simulink model "sampleModel1_pp_1_1"  (R2021b)
settings: Solver=VariableStepAuto  StartTime=0.0  StopTime=10.0  RelTol=1e-3
undefined symbols (not defined in the file or in its folder): DiscIntNeverNeededParam, Newton, Raphson
libraries: simulink x18, slpidlib x4
settings Model: Creator=user  LastModifiedBy=cemery

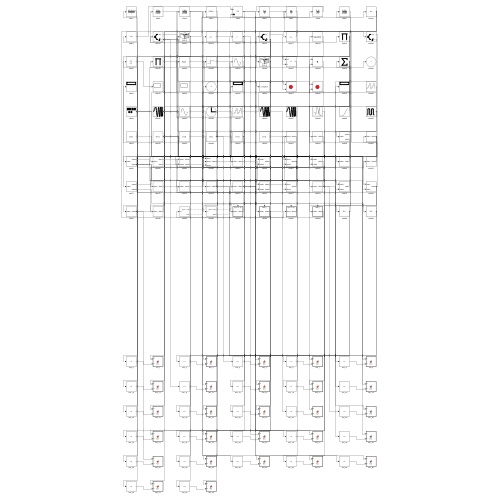
[thumbnail: Simulink's stored preview of the top-level diagram]
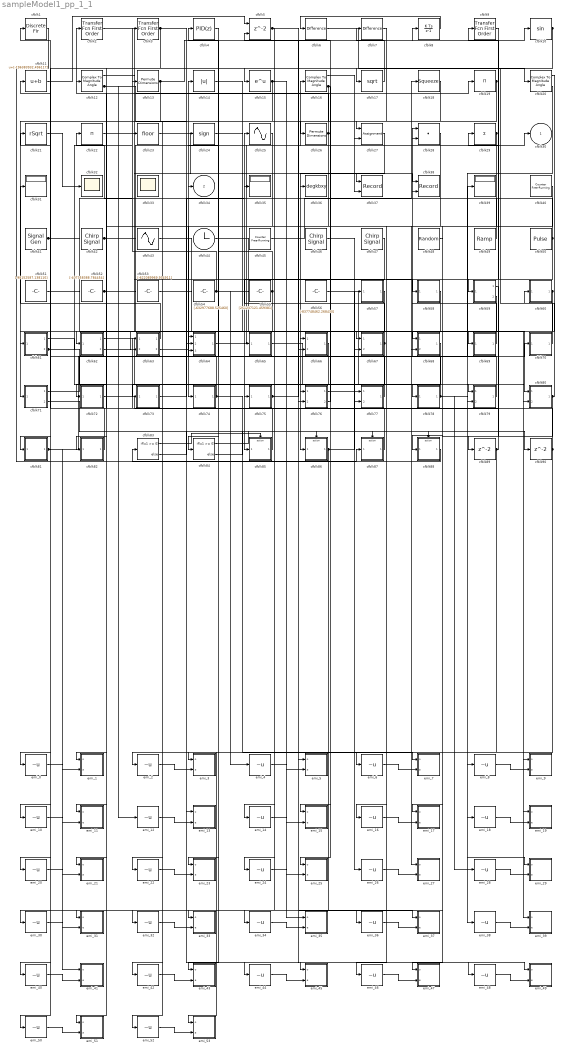
== system sampleModel1_pp_1_1 ==
  cfblk1 : DiscreteFir  SampleTime=1
  cfblk10 : Trigonometry
  cfblk11 : Bias  Bias=[-196383932.496117]
  cfblk12 : ComplexToMagnitudeAngle
  cfblk13 : PermuteDimensions
  cfblk14 : Abs
  cfblk15 : Math  SaturateOnIntegerOverflow=on
  cfblk16 : ComplexToMagnitudeAngle
  cfblk17 : Sqrt  SaturateOnIntegerOverflow=on
  cfblk18 : Squeeze
  cfblk19 : Product  Inputs=*
  cfblk2 : simulink/Discrete/Transfer Fcn First Order  PoleZ=0.95  ICPrevOutput=0.0  DoSatur=off
  cfblk20 : ComplexToMagnitudeAngle
  cfblk21 : Sqrt  Operator=rSqrt  AlgorithmType=Newton-Raphson  SaturateOnIntegerOverflow=on
  cfblk22 : Product  Inputs=*
  cfblk23 : Rounding
  cfblk24 : Signum
  cfblk25 : Sin  TimeSource=Use external signal  SampleTime=0
  cfblk26 : PermuteDimensions
  cfblk27 : Assignment  DiagnosticForDimensions=Warning  IndexOptions=Index vector (dialog)  Indices=1  OutputSizes=1
  cfblk28 : DotProduct  InputSameDT=on  OutDataTypeStr=Inherit: Inherit via internal rule
  cfblk29 : Sum  Inputs=+
  cfblk3 : simulink/Discrete/Transfer Fcn First Order  PoleZ=0.95  ICPrevOutput=0.0  DoSatur=off
  cfblk31 : Display
  cfblk32 : Scope
  cfblk33 : Scope
      settings: Floating=on
  cfblk35 : Display
  cfblk36 : ToWorkspace  VariableName=degkbxy  SaveFormat=Timeseries  SampleTime=-1
  cfblk37 : Record  FileSettingsInternal="{\"entries\":[{\"content\":{\"excelSettings\":{\"content\":{},\"type\":\"Streamout.ExcelSettings\"}},\"type\":\"Streamout.FileSettingStorage\",\"uuid\":\"343f84db-81de-408b-b1a6-f489dfd9fe13\"}],\"packageUris\":[\"http://schema.mathworks.com/mf0/streamout_blocks/R2020a\"],\"version\":\"1.0\"}"  Layout=[1 1]  SignalsInternal="{\"entries\":[{\"content\":{\"signals\":[{\"content\":{\"blockPath\":[\"sampleModel1_pp_1_1/cfblk37\"],\"channel\":[],\"dimensions\":[1],\"domain\":\"sampleModel1_pp_1_1/cfblk37\",\"lineColor\":\"#a2142f\",\"plots\":[],\"port\":1,\"sid\":[\"\"],\"signalID\":352,\"signalName\":\"cfblk14\"},\"type\":\"RecordBlkView.Signal\",\"uuid\":\"d3050f78-5135-48a5-bc90-ebe40b8d4c52\"},{\"content\":{\"blockPath\":[\"sampleModel1_pp_1_1/cfblk37\"],\"channel\":[],\"dimensions\":[1],\"domain\":\"sampleModel1_pp_1_1/cfblk37\",\"lineColor\":\"#139fff\",\"plots\":[],\"port\":2,\"sid\":[\"\"],\"signalID\":356,\"signalName\":\"cfblk16:1\"},\"type\":\"RecordBlkView.Signal\",\"uuid\":\"865a0524-d04f-4987-bc2a-acccf598b7a1\"}]},\"type\":\"RecordBlkView.InputSignals\",\"uuid\":\"039c24d2-93b4-4ea1-bba3-5a71198a0a0e\"}],\"packageUris\":[\"http://schema.mathworks.com/mf0/streamout_blocks/R2020a\"],\"version\":\"1.0\"}"  VisualizationBindings="{\"xyplotplugin\":{\"info\":[{\"series\":[],\"subplotID\":1}]}}"  CompatibilityTag=XY
  cfblk38 : Record  FileSettingsInternal="{\"entries\":[{\"content\":{\"excelSettings\":{\"content\":{},\"type\":\"Streamout.ExcelSettings\"}},\"type\":\"Streamout.FileSettingStorage\",\"uuid\":\"0a5133d1-d1dd-419a-b9c3-011ad09917cf\"}],\"packageUris\":[\"http://schema.mathworks.com/mf0/streamout_blocks/R2020a\"],\"version\":\"1.0\"}"  Layout=[1 1]  SignalsInternal="{\"entries\":[{\"content\":{\"signals\":[{\"content\":{\"blockPath\":[\"sampleModel1_pp_1_1/cfblk38\"],\"channel\":[],\"dimensions\":[1],\"domain\":\"sampleModel1_pp_1_1/cfblk38\",\"lineColor\":\"#ff6929\",\"plots\":[],\"port\":1,\"sid\":[\"\"],\"signalID\":360,\"signalName\":\"cfblk2\"},\"type\":\"RecordBlkView.Signal\",\"uuid\":\"c96adaa5-4d01-4fb0-8fa5-fc7ee38b0bf9\"},{\"content\":{\"blockPath\":[\"sampleModel1_pp_1_1/cfblk38\"],\"channel\":[],\"dimensions\":[1],\"domain\":\"sampleModel1_pp_1_1/cfblk38\",\"lineColor\":\"#b746ff\",\"plots\":[],\"port\":2,\"sid\":[\"\"],\"signalID\":364,\"signalName\":\"cfblk49\"},\"type\":\"RecordBlkView.Signal\",\"uuid\":\"90865e12-c543-48e7-a36c-e57c8157b30f\"}]},\"type\":\"RecordBlkView.InputSignals\",\"uuid\":\"fc363daa-8f32-40cf-99d0-3b294b312640\"}],\"packageUris\":[\"http://schema.mathworks.com/mf0/streamout_blocks/R2020a\"],\"version\":\"1.0\"}"  VisualizationBindings="{\"xyplotplugin\":{\"info\":[{\"series\":[],\"subplotID\":1}]}}"  CompatibilityTag=XY
  cfblk39 : Display
  cfblk4 : slpidlib/PID Controller  Controller=PID  Form=Parallel  TimeDomain=Discrete-time  UseExternalTs=off  SampleTime=1  IntegratorMethod=Forward Euler  FilterMethod=Forward Euler  ControllerParametersSource=internal  P=1  I=1  D=0  UseFilter=on  N=100  TunerSelectOption=Transfer Function Based (PID Tuner App)  InitialConditionSource=internal  InitialConditionForIntegrator=0  InitialConditionForFilter=0  DifferentiatorICPrevScaledInput=0  ExternalReset=none  TrackingMode=off  Kt=1  LimitOutput=off  SatLimitsSource=internal  UpperSaturationLimit=inf  LowerSaturationLimit=-inf  LinearizeAsGain=off  AntiWindupMode=none  Kb=1  POutMin=[]  POutMax=[]  IOutMin=[]  IOutMax=[]  DOutMin=[]  DOutMax=[]  NOutMin=[]  NOutMax=[]  SumOutMin=[]  SumOutMax=[]  SaturationOutMin=[]  SaturationOutMax=[]  PParamMin=[]  PParamMax=[]  IParamMin=[]  IParamMax=[]  DParamMin=[]  DParamMax=[]  NParamMin=[]  NParamMax=[]  KbParamMin=[]  KbParamMax=[]  KtParamMin=[]  KtParamMax=[]  KbOutMin=[]  KbOutMax=[]  KtOutMin=[]  KtOutMax=[]  IntegratorOutMin=[]  IntegratorOutMax=[]  FilterOutMin=[]  FilterOutMax=[]  SumI1OutMin=[]  SumI1OutMax=[]  SumI2OutMin=[]  SumI2OutMax=[]  SumI3OutMin=[]  SumI3OutMax=[]  SumI4OutMin=[]  SumI4OutMax=[]  SumDOutMin=[]  SumDOutMax=[]  DifferentiatorOutMin=[]  DifferentiatorOutMax=[]  FilterDiffOutCoefMin=[]  FilterDiffOutCoefMax=[]  ReciprocalOutMin=[]  ReciprocalOutMax=[]  SumDenOutMin=[]  SumDenOutMax=[]  SumNumOutMin=[]  SumNumOutMax=[]  DivideOutMin=[]  DivideOutMax=[]  UdiffTsProdOutMin=[]  UdiffTsProdOutMax=[]  NTsProdOutMin=[]  NTsProdOutMax=[]  UintegralTsProdOutMin=[]  UintegralTsProdOutMax=[]  UngainTsProdOutMin=[]  UngainTsProdOutMax=[]  IntegratorContinuousStateAttributes=''  IntegratorStateMustResolveToSignalObject=off  IntegratorRTWStateStorageClass=Auto  FilterContinuousStateAttributes=''  FilterStateMustResolveToSignalObject=off  FilterRTWStateStorageClass=Auto  ParallelPVariant=InternalParameters  IdealPVariant=Disabled  IVariant=InternalParameters  DVariant=InternalParameters  IntegratorVariant=Discrete  SatVariant=Disabled  AWVariant=Passthrough  PCopyVariant=Disabled  TRVariant=Disabled  FdbkBlocksVariant=Forward  IdealPFdbkVariant=Disabled  SatFdbkVariant=Disabled  DerivativeFilterVariant=ForwardEulerFilter  NVariant=InternalParameters  NCopyVariant=Disabled  FilterICVariant=InternalICsFilter  IntegratorICVariant=InternalICs  ExternalResetVariant=Disabled  TRSumVariant=Passthrough  SumFdbkVariant=Disabled  SumVariant=Sum_PID  TsampFilterVariant=InternalTs  TsampNgainVariant=Passthrough  TsampIntegralVariant=Passthrough  ExternalSaturationOutDataTypeStr=Inherit: Same as second input
  cfblk40 : simulink/Sources/Counter Free-Running  NumBits=[29.000000]  tsamp=-1
  cfblk41 : SignalGenerator  WaveForm=square  Amplitude=[-21494723.199962]
  cfblk42 : simulink/Sources/Chirp Signal  f1=[-261506437.759570]  T=[-777594489.412425]  f2=[560504136.642276]
  cfblk43 : Sin  Amplitude=[-220522326.077493]  Bias=[-516617428.172335]  SampleTime=0
  cfblk44 : Clock
  cfblk45 : simulink/Sources/Counter Free-Running  NumBits=[24.000000]  tsamp=-1
  cfblk46 : simulink/Sources/Chirp Signal  f1=[-807090949.663223]  T=[-736053414.787330]  f2=[884101181.550970]
  cfblk47 : simulink/Sources/Chirp Signal  f1=[912269080.459605]  T=[150417190.156931]  f2=[-880440914.105688]
  cfblk48 : RandomNumber  Mean=[-53044.017326]  Variance=[35315.857122]  Seed=[821194040.000000]  SampleTime=0.1
  cfblk49 : simulink/Sources/Ramp  slope=[-9691.931247]  start=[3.108166]  InitialOutput=[-662019.941075]
  cfblk5 : Delay  ShowEnablePort=on  SampleTime=1
      settings: InputPortMap=u0,e6
  cfblk50 : DiscretePulseGenerator  PulseType=Time based  Amplitude=[298230949.912904]  Period=[73172238.834145]  PulseWidth=5  PhaseDelay=[6.000000]
  cfblk51 : Constant  Value=[-98152587.138110]  SampleTime=1
  cfblk52 : Constant  Value=[-407358388.784454]  SampleTime=1
  cfblk53 : Constant  Value=[-622089969.934911]  SampleTime=1
  cfblk54 : Constant  Value=[-632977688.525460]  SampleTime=1
  cfblk55 : Constant  Value=[251237121.459381]  SampleTime=1
  cfblk56 : Constant  Value=[-837748462.268430]  SampleTime=1
  cfblk57 : Subsystem
  cfblk58 : Subsystem
  cfblk59 : Subsystem
  cfblk6 : simulink/Discrete/Difference  ICPrevInput=0.0  OutMin=[]  OutMax=[]  OutDataTypeStr=Inherit: Inherit via back propagation  OutDataType=fixdt(1, 16)  OutScaling=2^-10  DoSatur=off
  cfblk60 : Subsystem
  cfblk61 : Subsystem
  cfblk62 : Subsystem
  cfblk63 : Subsystem
  cfblk64 : Subsystem
  cfblk65 : Subsystem
  cfblk66 : Subsystem
  cfblk67 : Subsystem
  cfblk68 : Subsystem
  cfblk69 : Subsystem
  cfblk7 : simulink/Discrete/Difference  ICPrevInput=0.0  OutMin=[]  OutMax=[]  OutDataTypeStr=Inherit: Inherit via back propagation  OutDataType=fixdt(1, 16)  OutScaling=2^-10  DoSatur=off
  cfblk70 : Subsystem
  cfblk71 : Subsystem
  cfblk72 : Subsystem
  cfblk73 : Subsystem
  cfblk74 : Subsystem
  cfblk75 : Subsystem
  cfblk76 : Subsystem
  cfblk77 : Subsystem
  cfblk78 : Subsystem
  cfblk79 : Subsystem
  cfblk8 : DiscreteIntegrator  ICPrevOutput=DiscIntNeverNeededParam  ICPrevScaledInput=DiscIntNeverNeededParam
  cfblk80 : Subsystem
  cfblk81 : Subsystem
  cfblk82 : Subsystem
  cfblk83 : If  IfExpression=u1 >= 0  SampleTime=1
  cfblk84 : If  IfExpression=u1 >= 0  SampleTime=1
  cfblk85 : Subsystem  TreatAsAtomicUnit=on
  cfblk86 : Subsystem  TreatAsAtomicUnit=on
  cfblk87 : Subsystem  TreatAsAtomicUnit=on
  cfblk88 : Subsystem  TreatAsAtomicUnit=on
  cfblk89 : Delay  SampleTime=1
  cfblk9 : simulink/Discrete/Transfer Fcn First Order  PoleZ=0.95  ICPrevOutput=0.0  DoSatur=off
  cfblk90 : Delay  SampleTime=1
  emi_{0,2,4,6,8,10,12,14,16,18,20,22,24,26,28,30,32,34,36,38,40,42,44,46,48,50,52} (27 alike) : UnaryMinus
  emi_1 : MATLAB Function  TreatAsAtomicUnit=on
  emi_11 : MATLAB Function  TreatAsAtomicUnit=on
  emi_13 : MATLAB Function  TreatAsAtomicUnit=on
  emi_15 : MATLAB Function  TreatAsAtomicUnit=on
  emi_17 : MATLAB Function  TreatAsAtomicUnit=on
  emi_19 : MATLAB Function  TreatAsAtomicUnit=on
  emi_21 : MATLAB Function  TreatAsAtomicUnit=on
  emi_23 : MATLAB Function  TreatAsAtomicUnit=on
  emi_25 : MATLAB Function  TreatAsAtomicUnit=on
  emi_27 : MATLAB Function  TreatAsAtomicUnit=on
  emi_29 : MATLAB Function  TreatAsAtomicUnit=on
  emi_3 : MATLAB Function  TreatAsAtomicUnit=on
  emi_31 : MATLAB Function  TreatAsAtomicUnit=on
  emi_33 : MATLAB Function  TreatAsAtomicUnit=on
  emi_35 : MATLAB Function  TreatAsAtomicUnit=on
  emi_37 : MATLAB Function  TreatAsAtomicUnit=on
  emi_39 : MATLAB Function  TreatAsAtomicUnit=on
  emi_41 : MATLAB Function  TreatAsAtomicUnit=on
  emi_43 : MATLAB Function  TreatAsAtomicUnit=on
  emi_45 : MATLAB Function  TreatAsAtomicUnit=on
  emi_47 : MATLAB Function  TreatAsAtomicUnit=on
  emi_49 : MATLAB Function  TreatAsAtomicUnit=on
  emi_5 : MATLAB Function  TreatAsAtomicUnit=on
  emi_51 : MATLAB Function  TreatAsAtomicUnit=on
  emi_53 : MATLAB Function  TreatAsAtomicUnit=on
  emi_7 : MATLAB Function  TreatAsAtomicUnit=on
  emi_9 : MATLAB Function  TreatAsAtomicUnit=on
  cfblk30 : Outport
  cfblk34 : Outport  Port=2
  wires:
  cfblk19/1 -> cfblk71/1(cfblk1), emi_42/1, emi_43/1(o)
  cfblk63/1(cfblk2) -> cfblk31/1
  cfblk67/1(cfblk2) -> cfblk25/1, emi_22/1, emi_23/1(o)
  cfblk62/1(cfblk2) -> cfblk28/1
  cfblk44/1 -> cfblk68/1(cfblk1)
  cfblk26/1 -> cfblk2/1, emi_14/1, emi_15/1(o)
  cfblk21/1 -> cfblk32/1
  cfblk74/1(cfblk2) -> cfblk14/1, emi_6/1, emi_7/1(o)
  cfblk79/1(cfblk2) -> cfblk34/1
  cfblk69/1(cfblk2) -> cfblk28/2
  cfblk72/1(cfblk2) -> cfblk29/1
  cfblk29/1 -> cfblk74/1(cfblk1), emi_46/1, emi_47/1(o)
  cfblk70/1(cfblk2) -> cfblk15/1
  cfblk23/1 -> cfblk86/1(cfblk1)
  cfblk43/1 -> cfblk66/1(cfblk1)
  cfblk65/1(cfblk2) -> cfblk78/1(cfblk1)
  cfblk77/1(cfblk2) -> cfblk11/1
  cfblk48/1 -> cfblk88/1(cfblk1)
  cfblk53/1 -> cfblk80/1(cfblk1)
  cfblk13/1 -> cfblk10/1, emi_0/1, emi_1/1(o)
  cfblk64/1(cfblk2) -> cfblk30/1
  cfblk68/1(cfblk2) -> cfblk76/1(cfblk1)
  cfblk50/1 -> cfblk22/1, emi_16/1, emi_17/1(o)
  cfblk8/1 -> cfblk6/1
  cfblk12/1 -> cfblk58/1(cfblk1)
  cfblk9/1 -> cfblk59/1(cfblk1)
  cfblk78/1(cfblk2) -> cfblk4/1, emi_28/1, emi_29/1(o)
  cfblk85/1(cfblk2) -> cfblk63/1(cfblk1)
  cfblk52/1 -> cfblk69/1(cfblk1), emi_38/1, emi_39/1(o)
  cfblk76/1(cfblk2) -> cfblk77/1(cfblk1)
  cfblk1/1 -> cfblk87/1(cfblk1)
  cfblk56/1 -> cfblk79/1(cfblk1)
  cfblk47/1 -> cfblk85/1(cfblk1)
  cfblk71/1(cfblk2) -> cfblk39/1
  cfblk45/1 -> cfblk18/1
  cfblk51/1 -> cfblk80/2(cfblk3)
  cfblk62/2(cfblk4) -> cfblk76/2(cfblk4)
  cfblk15/1 -> cfblk62/1(cfblk1), emi_34/1, emi_35/1(o)
  cfblk5/1 -> cfblk65/1(cfblk1), emi_36/1, emi_37/1(o)
  cfblk59/2(cfblk3) -> cfblk63/2(cfblk4)
  cfblk81/1(cfblk2) -> cfblk70/1(cfblk1), emi_40/1, emi_41/1(o)
  cfblk66/1(cfblk2) -> cfblk84/1
  cfblk86/1(cfblk2) -> cfblk57/1(cfblk1), emi_30/1, emi_31/1(o)
  cfblk2/1 -> cfblk38/1
  cfblk75/1(cfblk2) -> cfblk8/1, emi_48/1, emi_49/1(o)
  cfblk73/1(cfblk2) -> cfblk35/1
  cfblk42/1 -> cfblk16/1, emi_8/1, emi_9/1(o)
  cfblk4/1 -> cfblk64/1(cfblk1)
  cfblk22/1 -> cfblk64/2(cfblk3)
  cfblk41/1 -> cfblk3/1, emi_26/1, emi_27/1(o)
  cfblk10/1 -> cfblk17/1, emi_10/1, emi_11/1(o)
  cfblk12/2 -> cfblk19/1, emi_12/1, emi_13/1(o)
  cfblk6/1 -> cfblk20/1
  cfblk20/1 -> cfblk67/1(cfblk1)
  cfblk58/1(cfblk2) -> cfblk61/1(cfblk1)
  cfblk49/1 -> cfblk38/2
  cfblk14/1 -> cfblk37/1
  cfblk80/1(cfblk2) -> cfblk60/1(cfblk1), emi_32/1, emi_33/1(o)
  cfblk20/2 -> cfblk79/2(cfblk3)
  cfblk54/1 -> cfblk13/1, emi_4/1, emi_5/1(o)
  cfblk28/1 -> cfblk68/2(cfblk5)
  cfblk87/1(cfblk2) -> cfblk21/1
  cfblk11/1 -> cfblk5/1
  cfblk17/1 -> cfblk7/1
  cfblk57/1(cfblk2) -> cfblk67/2(cfblk4)
  cfblk82/1(cfblk2) -> cfblk1/1
  cfblk61/1(cfblk2) -> cfblk75/1(cfblk1)
  cfblk88/1(cfblk2) -> cfblk83/1
  cfblk60/1(cfblk2) -> cfblk81/1(cfblk1), emi_50/1, emi_51/1(o)
  cfblk16/1 -> cfblk37/2
  cfblk7/1 -> cfblk27/1
  cfblk76/2(cfblk5) -> cfblk5/2
  cfblk18/1 -> cfblk27/2
  cfblk27/1 -> cfblk36/1
  cfblk3/1 -> cfblk72/1(cfblk1), emi_44/1, emi_45/1(o)
  cfblk46/1 -> cfblk77/2(cfblk4)
  cfblk25/1 -> cfblk73/1(cfblk1)
  cfblk16/2 -> cfblk26/1, emi_24/1, emi_25/1(o)
  cfblk61/2(cfblk3) -> cfblk23/1, emi_18/1, emi_19/1(o)
  cfblk63/2(cfblk5) -> cfblk64/3(cfblk4)
  cfblk55/1 -> cfblk24/1, emi_20/1, emi_21/1(o)
  cfblk40/1 -> cfblk82/1(cfblk1)
  cfblk24/1 -> cfblk66/2(cfblk5)
  cfblk83/1 -> cfblk85/Action
  cfblk83/2 -> cfblk86/Action
  cfblk84/1 -> cfblk87/Action
  cfblk84/2 -> cfblk88/Action
  cfblk59/1(cfblk2) -> cfblk89/1
  cfblk89/1 -> cfblk9/1, emi_52/1, emi_53/1(o)
  cfblk71/2(cfblk5) -> cfblk90/1
  cfblk90/1 -> cfblk12/1, emi_2/1, emi_3/1(o)
  emi_0/1 -> emi_1/2(e)
  emi_2/1 -> emi_3/2(e)
  emi_4/1 -> emi_5/2(e)
  emi_6/1 -> emi_7/2(e)
  emi_8/1 -> emi_9/2(e)
  emi_10/1 -> emi_11/2(e)
  emi_12/1 -> emi_13/2(e)
  emi_14/1 -> emi_15/2(e)
  emi_16/1 -> emi_17/2(e)
  emi_18/1 -> emi_19/2(e)
  emi_20/1 -> emi_21/2(e)
  emi_22/1 -> emi_23/2(e)
  emi_24/1 -> emi_25/2(e)
  emi_26/1 -> emi_27/2(e)
  emi_28/1 -> emi_29/2(e)
  emi_30/1 -> emi_31/2(e)
  emi_32/1 -> emi_33/2(e)
  emi_34/1 -> emi_35/2(e)
  emi_36/1 -> emi_37/2(e)
  emi_38/1 -> emi_39/2(e)
  emi_40/1 -> emi_41/2(e)
  emi_42/1 -> emi_43/2(e)
  emi_44/1 -> emi_45/2(e)
  emi_46/1 -> emi_47/2(e)
  emi_48/1 -> emi_49/2(e)
  emi_50/1 -> emi_51/2(e)
  emi_52/1 -> emi_53/2(e)

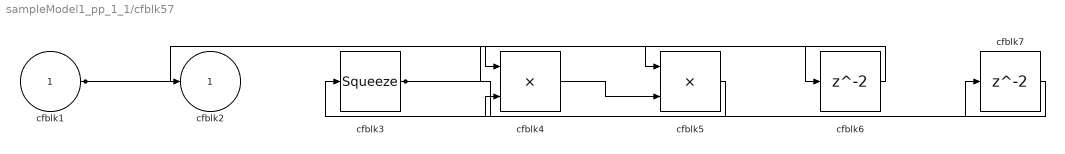
== system sampleModel1_pp_1_1/cfblk57 ==
  cfblk1 : Inport
  cfblk3 : Squeeze
  cfblk4 : Product
  cfblk5 : Product
  cfblk6 : Delay  SampleTime=1
  cfblk7 : Delay  SampleTime=1
  cfblk2 : Outport
  wires:
  cfblk3/1 -> cfblk6/1, cfblk7/1
  cfblk5/1 -> cfblk3/1
  cfblk1/1 -> cfblk4/1, cfblk2/1
  cfblk4/1 -> cfblk5/2
  cfblk6/1 -> cfblk5/1
  cfblk7/1 -> cfblk4/2

== system sampleModel1_pp_1_1/cfblk58 ==
  cfblk1 : Inport
  cfblk3 : DotProduct  InputSameDT=on  OutDataTypeStr=Inherit: Inherit via internal rule
  cfblk2 : Outport
  wires:
  cfblk1/1 -> cfblk3/1, cfblk3/2
  cfblk3/1 -> cfblk2/1

== system sampleModel1_pp_1_1/cfblk59 ==
  cfblk1 : Inport
  cfblk2 : Outport
  cfblk3 : Outport  Port=2
  wires:
  cfblk1/1 -> cfblk2/1, cfblk3/1

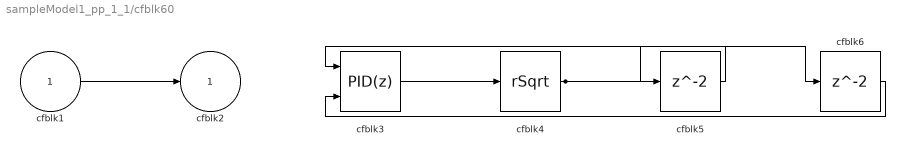
== system sampleModel1_pp_1_1/cfblk60 ==
  cfblk1 : Inport
  cfblk3 : slpidlib/PID Controller (2DOF)  Controller=PID  Form=Parallel  TimeDomain=Discrete-time  UseExternalTs=off  SampleTime=1  IntegratorMethod=Forward Euler  FilterMethod=Forward Euler  ControllerParametersSource=internal  P=1  I=1  D=0  UseFilter=on  N=100  b=1  c=1  TunerSelectOption=Transfer Function Based (PID Tuner App)  InitialConditionSource=internal  InitialConditionForIntegrator=0  InitialConditionForFilter=0  DifferentiatorICPrevScaledInput=0  ExternalReset=none  TrackingMode=off  Kt=1  LimitOutput=off  SatLimitsSource=internal  UpperSaturationLimit=inf  LowerSaturationLimit=-inf  LinearizeAsGain=off  AntiWindupMode=none  Kb=1  POutMin=[]  POutMax=[]  IOutMin=[]  IOutMax=[]  DOutMin=[]  DOutMax=[]  NOutMin=[]  NOutMax=[]  bOutMin=[]  bOutMax=[]  cOutMin=[]  cOutMax=[]  SumOutMin=[]  SumOutMax=[]  SaturationOutMin=[]  SaturationOutMax=[]  PParamMin=[]  PParamMax=[]  IParamMin=[]  IParamMax=[]  DParamMin=[]  DParamMax=[]  NParamMin=[]  NParamMax=[]  bParamMin=[]  bParamMax=[]  cParamMin=[]  cParamMax=[]  KbParamMin=[]  KbParamMax=[]  KtParamMin=[]  KtParamMax=[]  KbOutMin=[]  KbOutMax=[]  KtOutMin=[]  KtOutMax=[]  IntegratorOutMin=[]  IntegratorOutMax=[]  FilterOutMin=[]  FilterOutMax=[]  SumI1OutMin=[]  SumI1OutMax=[]  SumI2OutMin=[]  SumI2OutMax=[]  SumI3OutMin=[]  SumI3OutMax=[]  SumI4OutMin=[]  SumI4OutMax=[]  SumDOutMin=[]  SumDOutMax=[]  Sum1OutMin=[]  Sum1OutMax=[]  Sum2OutMin=[]  Sum2OutMax=[]  Sum3OutMin=[]  Sum3OutMax=[]  DifferentiatorOutMin=[]  DifferentiatorOutMax=[]  FilterDiffOutCoefMin=[]  FilterDiffOutCoefMax=[]  ReciprocalOutMin=[]  ReciprocalOutMax=[]  SumDenOutMin=[]  SumDenOutMax=[]  SumNumOutMin=[]  SumNumOutMax=[]  DivideOutMin=[]  DivideOutMax=[]  UdiffTsProdOutMin=[]  UdiffTsProdOutMax=[]  NTsProdOutMin=[]  NTsProdOutMax=[]  UintegralTsProdOutMin=[]  UintegralTsProdOutMax=[]  UngainTsProdOutMin=[]  UngainTsProdOutMax=[]  IntegratorContinuousStateAttributes=''  IntegratorStateMustResolveToSignalObject=off  IntegratorRTWStateStorageClass=Auto  FilterContinuousStateAttributes=''  FilterStateMustResolveToSignalObject=off  FilterRTWStateStorageClass=Auto  ParallelPVariant=InternalParameters  IdealPVariant=Disabled  IVariant=InternalParameters  DVariant=InternalParameters  bVariant=InternalParameters  cVariant=InternalParameters  IntegratorVariant=Discrete  SatVariant=Disabled  AWVariant=Passthrough  PCopyVariant=Disabled  TRVariant=Disabled  FdbkBlocksVariant=Forward  IdealPFdbkVariant=Disabled  SatFdbkVariant=Disabled  DerivativeFilterVariant=ForwardEulerFilter  NVariant=InternalParameters  NCopyVariant=Disabled  FilterICVariant=InternalICsFilter  IntegratorICVariant=InternalICs  ExternalResetVariant=Disabled  TRSumVariant=Passthrough  SumFdbkVariant=Disabled  SumVariant=Sum_PID  TsampFilterVariant=InternalTs  TsampNgainVariant=Passthrough  TsampIntegralVariant=Passthrough  ExternalSaturationOutDataTypeStr=Inherit: Same as second input
      settings: SourceProductBaseCode=SL
  cfblk4 : Sqrt  Operator=rSqrt  AlgorithmType=Newton-Raphson  SaturateOnIntegerOverflow=on
  cfblk5 : Delay  SampleTime=1
  cfblk6 : Delay  SampleTime=1
  cfblk2 : Outport
  wires:
  cfblk4/1 -> cfblk5/1, cfblk6/1
  cfblk1/1 -> cfblk2/1
  cfblk3/1 -> cfblk4/1
  cfblk5/1 -> cfblk3/1
  cfblk6/1 -> cfblk3/2

== system sampleModel1_pp_1_1/cfblk61 ==
  cfblk1 : Inport
  cfblk2 : Outport
  cfblk3 : Outport  Port=2
  wires:
  cfblk1/1 -> cfblk3/1, cfblk2/1

== system sampleModel1_pp_1_1/cfblk62 ==
  cfblk1 : Inport
  cfblk3 : Product
  cfblk2 : Outport
  cfblk4 : Outport  Port=2
  wires:
  cfblk1/1 -> cfblk2/1, cfblk3/1, cfblk3/2
  cfblk3/1 -> cfblk4/1

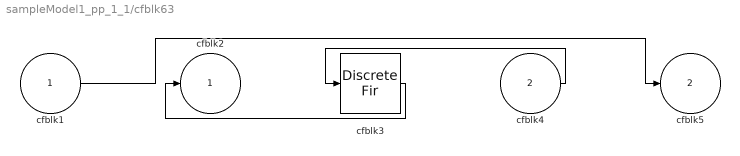
== system sampleModel1_pp_1_1/cfblk63 ==
  cfblk1 : Inport
  cfblk4 : Inport  Port=2
  cfblk3 : DiscreteFir  SampleTime=1
  cfblk2 : Outport
  cfblk5 : Outport  Port=2
  wires:
  cfblk4/1 -> cfblk3/1
  cfblk3/1 -> cfblk2/1
  cfblk1/1 -> cfblk5/1

== system sampleModel1_pp_1_1/cfblk64 ==
  cfblk1 : Inport
  cfblk3 : Inport  Port=2
  cfblk4 : Inport  Port=3
  cfblk2 : Outport
  wires:
  cfblk4/1 -> cfblk2/1

== system sampleModel1_pp_1_1/cfblk65 ==
  cfblk1 : Inport
  cfblk3 : Delay  SampleTime=1
  cfblk4 : Constant  Value=[488148520.734925]  SampleTime=1
  cfblk2 : Outport
  wires:
  cfblk4/1 -> cfblk2/1
  cfblk1/1 -> cfblk3/1

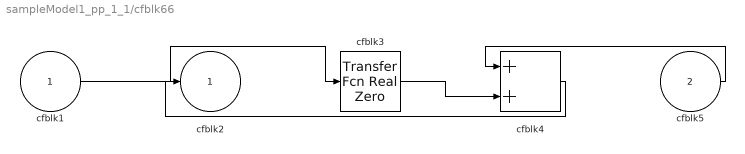
== system sampleModel1_pp_1_1/cfblk66 ==
  cfblk1 : Inport
  cfblk5 : Inport  Port=2
  cfblk3 : simulink/Discrete/Transfer Fcn Real Zero  ZeroZ=0.75  ICPrevInput=0.0  DoSatur=off
      settings: SourceProductBaseCode=SL
  cfblk4 : Sum
  cfblk2 : Outport
  wires:
  cfblk5/1 -> cfblk4/1
  cfblk1/1 -> cfblk3/1
  cfblk4/1 -> cfblk2/1
  cfblk3/1 -> cfblk4/2

== system sampleModel1_pp_1_1/cfblk67 ==
  cfblk1 : Inport
  cfblk4 : Inport  Port=2
  cfblk3 : simulink/Discrete/Transfer Fcn Lead or Lag  PoleZ=0.95  ZeroZ=0.75  ICPrevOutput=0.0  ICPrevInput=0.0  DoSatur=off
      settings: SourceProductBaseCode=SL
  cfblk2 : Outport
  wires:
  cfblk1/1 -> cfblk3/1
  cfblk4/1 -> cfblk2/1

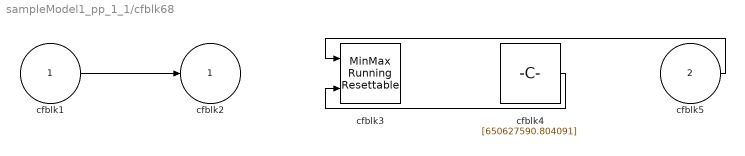
== system sampleModel1_pp_1_1/cfblk68 ==
  cfblk1 : Inport
  cfblk5 : Inport  Port=2
  cfblk3 : simulink/Math Operations/MinMax Running Resettable  Function=min  vinit=0.0
  cfblk4 : Constant  Value=[650627590.804091]  SampleTime=1
  cfblk2 : Outport
  wires:
  cfblk1/1 -> cfblk2/1
  cfblk5/1 -> cfblk3/1
  cfblk4/1 -> cfblk3/2

== system sampleModel1_pp_1_1/cfblk69 ==
  cfblk1 : Inport
  cfblk3 : Rounding
  cfblk4 : Reshape
  cfblk2 : Outport
  wires:
  cfblk3/1 -> cfblk2/1
  cfblk4/1 -> cfblk3/1
  cfblk1/1 -> cfblk4/1

== system sampleModel1_pp_1_1/cfblk70 ==
  cfblk1 : Inport
  cfblk3 : DiscreteFilter  SampleTime=1
  cfblk4 : UnaryMinus
  cfblk2 : Outport
  wires:
  cfblk1/1 -> cfblk4/1
  cfblk4/1 -> cfblk3/1
  cfblk3/1 -> cfblk2/1

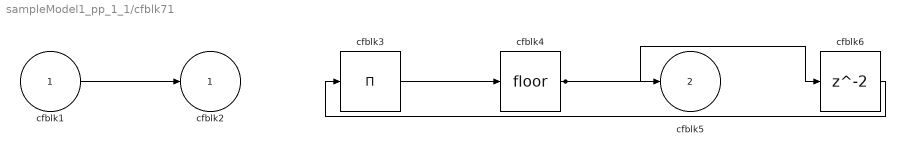
== system sampleModel1_pp_1_1/cfblk71 ==
  cfblk1 : Inport
  cfblk3 : Product  Inputs=*
  cfblk4 : Rounding
  cfblk6 : Delay  SampleTime=1
  cfblk2 : Outport
  cfblk5 : Outport  Port=2
  wires:
  cfblk3/1 -> cfblk4/1
  cfblk1/1 -> cfblk2/1
  cfblk4/1 -> cfblk5/1, cfblk6/1
  cfblk6/1 -> cfblk3/1

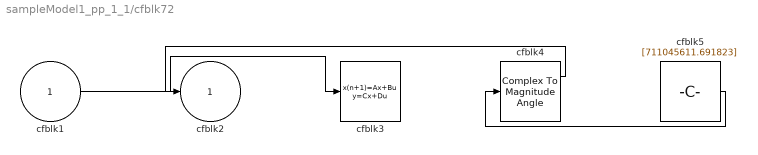
== system sampleModel1_pp_1_1/cfblk72 ==
  cfblk1 : Inport
  cfblk3 : DiscreteStateSpace
  cfblk4 : ComplexToMagnitudeAngle
  cfblk5 : Constant  Value=[711045611.691823]  SampleTime=1
  cfblk2 : Outport
  wires:
  cfblk1/1 -> cfblk3/1
  cfblk4/1 -> cfblk2/1
  cfblk5/1 -> cfblk4/1

== system sampleModel1_pp_1_1/cfblk73 ==
  cfblk1 : Inport
  cfblk3 : Gain  Gain=[234181768.786447]
  cfblk2 : Outport
  wires:
  cfblk3/1 -> cfblk2/1
  cfblk1/1 -> cfblk3/1

== system sampleModel1_pp_1_1/cfblk74 ==
  cfblk1 : Inport
  cfblk3 : UnitDelay  HasFrameUpgradeWarning=on
  cfblk4 : Sum  Inputs=|++
  cfblk2 : Outport
  wires:
  cfblk1/1 -> cfblk4/1, cfblk4/2
  cfblk4/1 -> cfblk3/1
  cfblk3/1 -> cfblk2/1

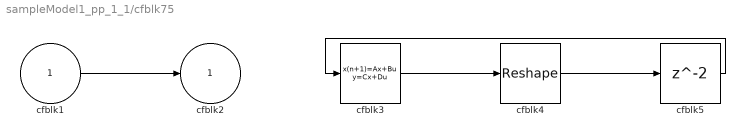
== system sampleModel1_pp_1_1/cfblk75 ==
  cfblk1 : Inport
  cfblk3 : DiscreteStateSpace
  cfblk4 : Reshape
  cfblk5 : Delay  SampleTime=1
  cfblk2 : Outport
  wires:
  cfblk1/1 -> cfblk2/1
  cfblk3/1 -> cfblk4/1
  cfblk4/1 -> cfblk5/1
  cfblk5/1 -> cfblk3/1

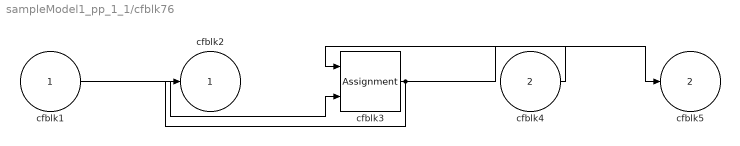
== system sampleModel1_pp_1_1/cfblk76 ==
  cfblk1 : Inport
  cfblk4 : Inport  Port=2
  cfblk3 : Assignment  DiagnosticForDimensions=Warning  IndexOptions=Index vector (dialog)  Indices=1  OutputSizes=1
  cfblk2 : Outport
  cfblk5 : Outport  Port=2
  wires:
  cfblk4/1 -> cfblk3/1
  cfblk1/1 -> cfblk3/2
  cfblk3/1 -> cfblk2/1, cfblk5/1

== system sampleModel1_pp_1_1/cfblk77 ==
  cfblk1 : Inport
  cfblk4 : Inport  Port=2
  cfblk3 : Product
  cfblk2 : Outport
  wires:
  cfblk4/1 -> cfblk3/1
  cfblk1/1 -> cfblk3/2
  cfblk3/1 -> cfblk2/1

== system sampleModel1_pp_1_1/cfblk78 ==
  cfblk1 : Inport
  cfblk3 : simulink/Discrete/Transfer Fcn Lead or Lag  PoleZ=0.95  ZeroZ=0.75  ICPrevOutput=0.0  ICPrevInput=0.0  DoSatur=off
      settings: SourceProductBaseCode=SL
  cfblk4 : Math  Operator=mod  SaturateOnIntegerOverflow=on
  cfblk5 : Constant  Value=[350664131.493999]  SampleTime=1
  cfblk2 : Outport
  wires:
  cfblk4/1 -> cfblk3/1
  cfblk1/1 -> cfblk4/1
  cfblk3/1 -> cfblk2/1
  cfblk5/1 -> cfblk4/2

== system sampleModel1_pp_1_1/cfblk79 ==
  cfblk1 : Inport
  cfblk3 : Inport  Port=2
  cfblk2 : Outport
  wires:
  cfblk1/1 -> cfblk2/1

== system sampleModel1_pp_1_1/cfblk80 ==
  cfblk1 : Inport
  cfblk3 : Inport  Port=2
  cfblk2 : Outport
  wires:
  cfblk1/1 -> cfblk2/1

== system sampleModel1_pp_1_1/cfblk81 ==
  cfblk1 : Inport
  cfblk3 : simulink/Discrete/Tapped Delay  vinit=0.0  samptime=-1  NumDelays=1  DelayOrder=Oldest  includeCurrent=off
  cfblk4 : DotProduct  InputSameDT=on  OutDataTypeStr=Inherit: Inherit via internal rule
  cfblk2 : Outport
  wires:
  cfblk4/1 -> cfblk2/1
  cfblk1/1 -> cfblk3/1
  cfblk3/1 -> cfblk4/1, cfblk4/2

== system sampleModel1_pp_1_1/cfblk82 ==
  cfblk1 : Inport
  cfblk3 : Constant  Value=[358033508.186404]  SampleTime=1
  cfblk4 : Constant  Value=[890348226.218803]  SampleTime=1
  cfblk2 : Outport
  wires:
  cfblk1/1 -> cfblk2/1

== system sampleModel1_pp_1_1/cfblk85 ==
  cfblk1 : Inport
  Action Port : ActionPort  ActionPortLabel=if(u1 >= 0)
  cfblk3 : simulink/Math Operations/Slider Gain  gain=1  low=0  high=2
  cfblk4 : Constant  Value=[-299563973.117790]  SampleTime=1
  cfblk2 : Outport
  wires:
  cfblk4/1 -> cfblk2/1
  cfblk1/1 -> cfblk3/1

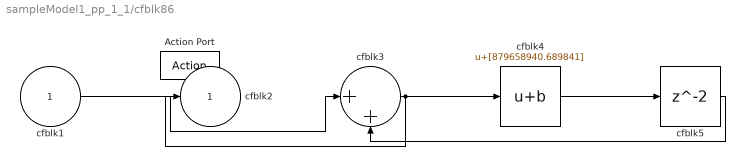
== system sampleModel1_pp_1_1/cfblk86 ==
  cfblk1 : Inport
  Action Port : ActionPort  ActionPortLabel=else
  cfblk3 : Sum  Inputs=|++
  cfblk4 : Bias  Bias=[879658940.689841]
  cfblk5 : Delay
  cfblk2 : Outport
  wires:
  cfblk1/1 -> cfblk3/1
  cfblk3/1 -> cfblk4/1, cfblk2/1
  cfblk4/1 -> cfblk5/1
  cfblk5/1 -> cfblk3/2

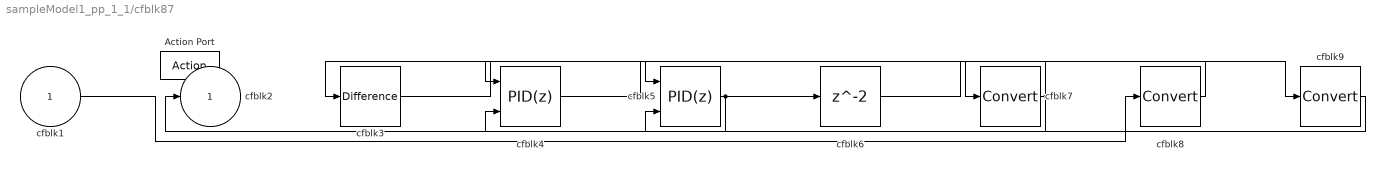
== system sampleModel1_pp_1_1/cfblk87 ==
  cfblk1 : Inport
  Action Port : ActionPort  ActionPortLabel=if(u1 >= 0)
  cfblk3 : simulink/Discrete/Difference  ICPrevInput=0.0  OutMin=[]  OutMax=[]  OutDataTypeStr=Inherit: Inherit via back propagation  OutDataType=fixdt(1, 16)  OutScaling=2^-10  DoSatur=off
  cfblk4 : slpidlib/PID Controller (2DOF)  Controller=PID  Form=Parallel  TimeDomain=Discrete-time  UseExternalTs=off  SampleTime=-1  IntegratorMethod=Forward Euler  FilterMethod=Forward Euler  ControllerParametersSource=internal  P=1  I=1  D=0  UseFilter=on  N=100  b=1  c=1  TunerSelectOption=Transfer Function Based (PID Tuner App)  InitialConditionSource=internal  InitialConditionForIntegrator=0  InitialConditionForFilter=0  DifferentiatorICPrevScaledInput=0  ExternalReset=none  TrackingMode=off  Kt=1  LimitOutput=off  SatLimitsSource=internal  UpperSaturationLimit=inf  LowerSaturationLimit=-inf  LinearizeAsGain=off  AntiWindupMode=none  Kb=1  POutMin=[]  POutMax=[]  IOutMin=[]  IOutMax=[]  DOutMin=[]  DOutMax=[]  NOutMin=[]  NOutMax=[]  bOutMin=[]  bOutMax=[]  cOutMin=[]  cOutMax=[]  SumOutMin=[]  SumOutMax=[]  SaturationOutMin=[]  SaturationOutMax=[]  PParamMin=[]  PParamMax=[]  IParamMin=[]  IParamMax=[]  DParamMin=[]  DParamMax=[]  NParamMin=[]  NParamMax=[]  bParamMin=[]  bParamMax=[]  cParamMin=[]  cParamMax=[]  KbParamMin=[]  KbParamMax=[]  KtParamMin=[]  KtParamMax=[]  KbOutMin=[]  KbOutMax=[]  KtOutMin=[]  KtOutMax=[]  IntegratorOutMin=[]  IntegratorOutMax=[]  FilterOutMin=[]  FilterOutMax=[]  SumI1OutMin=[]  SumI1OutMax=[]  SumI2OutMin=[]  SumI2OutMax=[]  SumI3OutMin=[]  SumI3OutMax=[]  SumI4OutMin=[]  SumI4OutMax=[]  SumDOutMin=[]  SumDOutMax=[]  Sum1OutMin=[]  Sum1OutMax=[]  Sum2OutMin=[]  Sum2OutMax=[]  Sum3OutMin=[]  Sum3OutMax=[]  DifferentiatorOutMin=[]  DifferentiatorOutMax=[]  FilterDiffOutCoefMin=[]  FilterDiffOutCoefMax=[]  ReciprocalOutMin=[]  ReciprocalOutMax=[]  SumDenOutMin=[]  SumDenOutMax=[]  SumNumOutMin=[]  SumNumOutMax=[]  DivideOutMin=[]  DivideOutMax=[]  UdiffTsProdOutMin=[]  UdiffTsProdOutMax=[]  NTsProdOutMin=[]  NTsProdOutMax=[]  UintegralTsProdOutMin=[]  UintegralTsProdOutMax=[]  UngainTsProdOutMin=[]  UngainTsProdOutMax=[]  IntegratorContinuousStateAttributes=''  IntegratorStateMustResolveToSignalObject=off  IntegratorRTWStateStorageClass=Auto  FilterContinuousStateAttributes=''  FilterStateMustResolveToSignalObject=off  FilterRTWStateStorageClass=Auto  ParallelPVariant=InternalParameters  IdealPVariant=Disabled  IVariant=InternalParameters  DVariant=InternalParameters  bVariant=InternalParameters  cVariant=InternalParameters  IntegratorVariant=Discrete  SatVariant=Disabled  AWVariant=Passthrough  PCopyVariant=Disabled  TRVariant=Disabled  FdbkBlocksVariant=Forward  IdealPFdbkVariant=Disabled  SatFdbkVariant=Disabled  DerivativeFilterVariant=ForwardEulerFilter  NVariant=InternalParameters  NCopyVariant=Disabled  FilterICVariant=InternalICsFilter  IntegratorICVariant=InternalICs  ExternalResetVariant=Disabled  TRSumVariant=Passthrough  SumFdbkVariant=Disabled  SumVariant=Sum_PID  TsampFilterVariant=InternalTs  TsampNgainVariant=Passthrough  TsampIntegralVariant=Passthrough  ExternalSaturationOutDataTypeStr=Inherit: Same as second input
      settings: SourceProductBaseCode=SL
  cfblk5 : slpidlib/PID Controller (2DOF)  Controller=PID  Form=Parallel  TimeDomain=Discrete-time  UseExternalTs=off  SampleTime=-1  IntegratorMethod=Forward Euler  FilterMethod=Forward Euler  ControllerParametersSource=internal  P=1  I=1  D=0  UseFilter=on  N=100  b=1  c=1  TunerSelectOption=Transfer Function Based (PID Tuner App)  InitialConditionSource=internal  InitialConditionForIntegrator=0  InitialConditionForFilter=0  DifferentiatorICPrevScaledInput=0  ExternalReset=none  TrackingMode=off  Kt=1  LimitOutput=off  SatLimitsSource=internal  UpperSaturationLimit=inf  LowerSaturationLimit=-inf  LinearizeAsGain=off  AntiWindupMode=none  Kb=1  POutMin=[]  POutMax=[]  IOutMin=[]  IOutMax=[]  DOutMin=[]  DOutMax=[]  NOutMin=[]  NOutMax=[]  bOutMin=[]  bOutMax=[]  cOutMin=[]  cOutMax=[]  SumOutMin=[]  SumOutMax=[]  SaturationOutMin=[]  SaturationOutMax=[]  PParamMin=[]  PParamMax=[]  IParamMin=[]  IParamMax=[]  DParamMin=[]  DParamMax=[]  NParamMin=[]  NParamMax=[]  bParamMin=[]  bParamMax=[]  cParamMin=[]  cParamMax=[]  KbParamMin=[]  KbParamMax=[]  KtParamMin=[]  KtParamMax=[]  KbOutMin=[]  KbOutMax=[]  KtOutMin=[]  KtOutMax=[]  IntegratorOutMin=[]  IntegratorOutMax=[]  FilterOutMin=[]  FilterOutMax=[]  SumI1OutMin=[]  SumI1OutMax=[]  SumI2OutMin=[]  SumI2OutMax=[]  SumI3OutMin=[]  SumI3OutMax=[]  SumI4OutMin=[]  SumI4OutMax=[]  SumDOutMin=[]  SumDOutMax=[]  Sum1OutMin=[]  Sum1OutMax=[]  Sum2OutMin=[]  Sum2OutMax=[]  Sum3OutMin=[]  Sum3OutMax=[]  DifferentiatorOutMin=[]  DifferentiatorOutMax=[]  FilterDiffOutCoefMin=[]  FilterDiffOutCoefMax=[]  ReciprocalOutMin=[]  ReciprocalOutMax=[]  SumDenOutMin=[]  SumDenOutMax=[]  SumNumOutMin=[]  SumNumOutMax=[]  DivideOutMin=[]  DivideOutMax=[]  UdiffTsProdOutMin=[]  UdiffTsProdOutMax=[]  NTsProdOutMin=[]  NTsProdOutMax=[]  UintegralTsProdOutMin=[]  UintegralTsProdOutMax=[]  UngainTsProdOutMin=[]  UngainTsProdOutMax=[]  IntegratorContinuousStateAttributes=''  IntegratorStateMustResolveToSignalObject=off  IntegratorRTWStateStorageClass=Auto  FilterContinuousStateAttributes=''  FilterStateMustResolveToSignalObject=off  FilterRTWStateStorageClass=Auto  ParallelPVariant=InternalParameters  IdealPVariant=Disabled  IVariant=InternalParameters  DVariant=InternalParameters  bVariant=InternalParameters  cVariant=InternalParameters  IntegratorVariant=Discrete  SatVariant=Disabled  AWVariant=Passthrough  PCopyVariant=Disabled  TRVariant=Disabled  FdbkBlocksVariant=Forward  IdealPFdbkVariant=Disabled  SatFdbkVariant=Disabled  DerivativeFilterVariant=ForwardEulerFilter  NVariant=InternalParameters  NCopyVariant=Disabled  FilterICVariant=InternalICsFilter  IntegratorICVariant=InternalICs  ExternalResetVariant=Disabled  TRSumVariant=Passthrough  SumFdbkVariant=Disabled  SumVariant=Sum_PID  TsampFilterVariant=InternalTs  TsampNgainVariant=Passthrough  TsampIntegralVariant=Passthrough  ExternalSaturationOutDataTypeStr=Inherit: Same as second input
      settings: SourceProductBaseCode=SL
  cfblk6 : Delay
  cfblk7 : DataTypeConversion
  cfblk8 : DataTypeConversion
  cfblk9 : DataTypeConversion
  cfblk2 : Outport
  wires:
  cfblk3/1 -> cfblk5/1
  cfblk4/1 -> cfblk7/1
  cfblk5/1 -> cfblk2/1, cfblk6/1
  cfblk7/1 -> cfblk3/1, cfblk5/2
  cfblk1/1 -> cfblk8/1
  cfblk8/1 -> cfblk4/1
  cfblk6/1 -> cfblk9/1
  cfblk9/1 -> cfblk4/2

== system sampleModel1_pp_1_1/cfblk88 ==
  cfblk1 : Inport
  Action Port : ActionPort  ActionPortLabel=else
  cfblk3 : Sin  TimeSource=Use external signal  SampleTime=0
  cfblk4 : Constant  Value=[40104934.780774]  SampleTime=1
  cfblk2 : Outport
  wires:
  cfblk3/1 -> cfblk2/1
  cfblk1/1 -> cfblk3/1

== matlab function sampleModel1_pp_1_1/emi_29 ==
  data: o input; e input
function  fcn(o, e)
o_inv = o^-1;
e_inv = e^-1;

emsg = 'sampleModel1_pp_1_1/emi_29';
 
if(o == e)
    assert(o_inv == e_inv, [emsg ' ; o_inv~=e_inv']);
    return;
end
 
if(o_inv > 0)
    assert(e_inv < 0, [emsg ' ; e_inv>=0']);
else
    assert(e_inv > 0, [emsg ' ; e_inv<=0']);
end

== matlab function sampleModel1_pp_1_1/emi_31 ==
  data: o input; e input
function  fcn(o, e)
o_inv = o^-1;
e_inv = e^-1;

emsg = 'sampleModel1_pp_1_1/emi_31';
 
if(o == e)
    assert(o_inv == e_inv, [emsg ' ; o_inv~=e_inv']);
    return;
end
 
if(o_inv > 0)
    assert(e_inv < 0, [emsg ' ; e_inv>=0']);
else
    assert(e_inv > 0, [emsg ' ; e_inv<=0']);
end

== matlab function sampleModel1_pp_1_1/emi_33 ==
  data: o input; e input
function  fcn(o, e)
o_inv = o^-1;
e_inv = e^-1;

emsg = 'sampleModel1_pp_1_1/emi_33';
 
if(o == e)
    assert(o_inv == e_inv, [emsg ' ; o_inv~=e_inv']);
    return;
end
 
if(o_inv > 0)
    assert(e_inv < 0, [emsg ' ; e_inv>=0']);
else
    assert(e_inv > 0, [emsg ' ; e_inv<=0']);
end

== matlab function sampleModel1_pp_1_1/emi_35 ==
  data: o input; e input
function  fcn(o, e)
o_inv = o^-1;
e_inv = e^-1;

emsg = 'sampleModel1_pp_1_1/emi_35';
 
if(o == e)
    assert(o_inv == e_inv, [emsg ' ; o_inv~=e_inv']);
    return;
end
 
if(o_inv > 0)
    assert(e_inv < 0, [emsg ' ; e_inv>=0']);
else
    assert(e_inv > 0, [emsg ' ; e_inv<=0']);
end

== matlab function sampleModel1_pp_1_1/emi_37 ==
  data: o input; e input
function  fcn(o, e)
o_inv = o^-1;
e_inv = e^-1;

emsg = 'sampleModel1_pp_1_1/emi_37';
 
if(o == e)
    assert(o_inv == e_inv, [emsg ' ; o_inv~=e_inv']);
    return;
end
 
if(o_inv > 0)
    assert(e_inv < 0, [emsg ' ; e_inv>=0']);
else
    assert(e_inv > 0, [emsg ' ; e_inv<=0']);
end

== matlab function sampleModel1_pp_1_1/emi_39 ==
  data: o input; e input
function  fcn(o, e)
o_inv = o^-1;
e_inv = e^-1;

emsg = 'sampleModel1_pp_1_1/emi_39';
 
if(o == e)
    assert(o_inv == e_inv, [emsg ' ; o_inv~=e_inv']);
    return;
end
 
if(o_inv > 0)
    assert(e_inv < 0, [emsg ' ; e_inv>=0']);
else
    assert(e_inv > 0, [emsg ' ; e_inv<=0']);
end

== matlab function sampleModel1_pp_1_1/emi_41 ==
  data: o input; e input
function  fcn(o, e)
o_inv = o^-1;
e_inv = e^-1;

emsg = 'sampleModel1_pp_1_1/emi_41';
 
if(o == e)
    assert(o_inv == e_inv, [emsg ' ; o_inv~=e_inv']);
    return;
end
 
if(o_inv > 0)
    assert(e_inv < 0, [emsg ' ; e_inv>=0']);
else
    assert(e_inv > 0, [emsg ' ; e_inv<=0']);
end

== matlab function sampleModel1_pp_1_1/emi_1 ==
  data: o input; e input
function  fcn(o, e)
o_inv = o^-1;
e_inv = e^-1;

emsg = 'sampleModel1_pp_1_1/emi_1';
 
if(o == e)
    assert(o_inv == e_inv, [emsg ' ; o_inv~=e_inv']);
    return;
end
 
if(o_inv > 0)
    assert(e_inv < 0, [emsg ' ; e_inv>=0']);
else
    assert(e_inv > 0, [emsg ' ; e_inv<=0']);
end

== matlab function sampleModel1_pp_1_1/emi_43 ==
  data: o input; e input
function  fcn(o, e)
o_inv = o^-1;
e_inv = e^-1;

emsg = 'sampleModel1_pp_1_1/emi_43';
 
if(o == e)
    assert(o_inv == e_inv, [emsg ' ; o_inv~=e_inv']);
    return;
end
 
if(o_inv > 0)
    assert(e_inv < 0, [emsg ' ; e_inv>=0']);
else
    assert(e_inv > 0, [emsg ' ; e_inv<=0']);
end

== matlab function sampleModel1_pp_1_1/emi_45 ==
  data: o input; e input
function  fcn(o, e)
o_inv = o^-1;
e_inv = e^-1;

emsg = 'sampleModel1_pp_1_1/emi_45';
 
if(o == e)
    assert(o_inv == e_inv, [emsg ' ; o_inv~=e_inv']);
    return;
end
 
if(o_inv > 0)
    assert(e_inv < 0, [emsg ' ; e_inv>=0']);
else
    assert(e_inv > 0, [emsg ' ; e_inv<=0']);
end

== matlab function sampleModel1_pp_1_1/emi_47 ==
  data: o input; e input
function  fcn(o, e)
o_inv = o^-1;
e_inv = e^-1;

emsg = 'sampleModel1_pp_1_1/emi_47';
 
if(o == e)
    assert(o_inv == e_inv, [emsg ' ; o_inv~=e_inv']);
    return;
end
 
if(o_inv > 0)
    assert(e_inv < 0, [emsg ' ; e_inv>=0']);
else
    assert(e_inv > 0, [emsg ' ; e_inv<=0']);
end

== matlab function sampleModel1_pp_1_1/emi_49 ==
  data: o input; e input
function  fcn(o, e)
o_inv = o^-1;
e_inv = e^-1;

emsg = 'sampleModel1_pp_1_1/emi_49';
 
if(o == e)
    assert(o_inv == e_inv, [emsg ' ; o_inv~=e_inv']);
    return;
end
 
if(o_inv > 0)
    assert(e_inv < 0, [emsg ' ; e_inv>=0']);
else
    assert(e_inv > 0, [emsg ' ; e_inv<=0']);
end

== matlab function sampleModel1_pp_1_1/emi_51 ==
  data: o input; e input
function  fcn(o, e)
o_inv = o^-1;
e_inv = e^-1;

emsg = 'sampleModel1_pp_1_1/emi_51';
 
if(o == e)
    assert(o_inv == e_inv, [emsg ' ; o_inv~=e_inv']);
    return;
end
 
if(o_inv > 0)
    assert(e_inv < 0, [emsg ' ; e_inv>=0']);
else
    assert(e_inv > 0, [emsg ' ; e_inv<=0']);
end

== matlab function sampleModel1_pp_1_1/emi_53 ==
  data: o input; e input
function  fcn(o, e)
o_inv = o^-1;
e_inv = e^-1;

emsg = 'sampleModel1_pp_1_1/emi_53';
 
if(o == e)
    assert(o_inv == e_inv, [emsg ' ; o_inv~=e_inv']);
    return;
end
 
if(o_inv > 0)
    assert(e_inv < 0, [emsg ' ; e_inv>=0']);
else
    assert(e_inv > 0, [emsg ' ; e_inv<=0']);
end

== matlab function sampleModel1_pp_1_1/emi_5 ==
  data: o input; e input
function  fcn(o, e)
o_inv = o^-1;
e_inv = e^-1;

emsg = 'sampleModel1_pp_1_1/emi_5';
 
if(o == e)
    assert(o_inv == e_inv, [emsg ' ; o_inv~=e_inv']);
    return;
end
 
if(o_inv > 0)
    assert(e_inv < 0, [emsg ' ; e_inv>=0']);
else
    assert(e_inv > 0, [emsg ' ; e_inv<=0']);
end

== matlab function sampleModel1_pp_1_1/emi_7 ==
  data: o input; e input
function  fcn(o, e)
o_inv = o^-1;
e_inv = e^-1;

emsg = 'sampleModel1_pp_1_1/emi_7';
 
if(o == e)
    assert(o_inv == e_inv, [emsg ' ; o_inv~=e_inv']);
    return;
end
 
if(o_inv > 0)
    assert(e_inv < 0, [emsg ' ; e_inv>=0']);
else
    assert(e_inv > 0, [emsg ' ; e_inv<=0']);
end

== matlab function sampleModel1_pp_1_1/emi_9 ==
  data: o input; e input
function  fcn(o, e)
o_inv = o^-1;
e_inv = e^-1;

emsg = 'sampleModel1_pp_1_1/emi_9';
 
if(o == e)
    assert(o_inv == e_inv, [emsg ' ; o_inv~=e_inv']);
    return;
end
 
if(o_inv > 0)
    assert(e_inv < 0, [emsg ' ; e_inv>=0']);
else
    assert(e_inv > 0, [emsg ' ; e_inv<=0']);
end

== matlab function sampleModel1_pp_1_1/emi_11 ==
  data: o input; e input
function  fcn(o, e)
o_inv = o^-1;
e_inv = e^-1;

emsg = 'sampleModel1_pp_1_1/emi_11';
 
if(o == e)
    assert(o_inv == e_inv, [emsg ' ; o_inv~=e_inv']);
    return;
end
 
if(o_inv > 0)
    assert(e_inv < 0, [emsg ' ; e_inv>=0']);
else
    assert(e_inv > 0, [emsg ' ; e_inv<=0']);
end

== matlab function sampleModel1_pp_1_1/emi_13 ==
  data: o input; e input
function  fcn(o, e)
o_inv = o^-1;
e_inv = e^-1;

emsg = 'sampleModel1_pp_1_1/emi_13';
 
if(o == e)
    assert(o_inv == e_inv, [emsg ' ; o_inv~=e_inv']);
    return;
end
 
if(o_inv > 0)
    assert(e_inv < 0, [emsg ' ; e_inv>=0']);
else
    assert(e_inv > 0, [emsg ' ; e_inv<=0']);
end

== matlab function sampleModel1_pp_1_1/emi_15 ==
  data: o input; e input
function  fcn(o, e)
o_inv = o^-1;
e_inv = e^-1;

emsg = 'sampleModel1_pp_1_1/emi_15';
 
if(o == e)
    assert(o_inv == e_inv, [emsg ' ; o_inv~=e_inv']);
    return;
end
 
if(o_inv > 0)
    assert(e_inv < 0, [emsg ' ; e_inv>=0']);
else
    assert(e_inv > 0, [emsg ' ; e_inv<=0']);
end

== matlab function sampleModel1_pp_1_1/emi_17 ==
  data: o input; e input
function  fcn(o, e)
o_inv = o^-1;
e_inv = e^-1;

emsg = 'sampleModel1_pp_1_1/emi_17';
 
if(o == e)
    assert(o_inv == e_inv, [emsg ' ; o_inv~=e_inv']);
    return;
end
 
if(o_inv > 0)
    assert(e_inv < 0, [emsg ' ; e_inv>=0']);
else
    assert(e_inv > 0, [emsg ' ; e_inv<=0']);
end

== matlab function sampleModel1_pp_1_1/emi_19 ==
  data: o input; e input
function  fcn(o, e)
o_inv = o^-1;
e_inv = e^-1;

emsg = 'sampleModel1_pp_1_1/emi_19';
 
if(o == e)
    assert(o_inv == e_inv, [emsg ' ; o_inv~=e_inv']);
    return;
end
 
if(o_inv > 0)
    assert(e_inv < 0, [emsg ' ; e_inv>=0']);
else
    assert(e_inv > 0, [emsg ' ; e_inv<=0']);
end

== matlab function sampleModel1_pp_1_1/emi_21 ==
  data: o input; e input
function  fcn(o, e)
o_inv = o^-1;
e_inv = e^-1;

emsg = 'sampleModel1_pp_1_1/emi_21';
 
if(o == e)
    assert(o_inv == e_inv, [emsg ' ; o_inv~=e_inv']);
    return;
end
 
if(o_inv > 0)
    assert(e_inv < 0, [emsg ' ; e_inv>=0']);
else
    assert(e_inv > 0, [emsg ' ; e_inv<=0']);
end

== matlab function sampleModel1_pp_1_1/emi_3 ==
  data: o input; e input
function  fcn(o, e)
o_inv = o^-1;
e_inv = e^-1;

emsg = 'sampleModel1_pp_1_1/emi_3';
 
if(o == e)
    assert(o_inv == e_inv, [emsg ' ; o_inv~=e_inv']);
    return;
end
 
if(o_inv > 0)
    assert(e_inv < 0, [emsg ' ; e_inv>=0']);
else
    assert(e_inv > 0, [emsg ' ; e_inv<=0']);
end

== matlab function sampleModel1_pp_1_1/emi_23 ==
  data: o input; e input
function  fcn(o, e)
o_inv = o^-1;
e_inv = e^-1;

emsg = 'sampleModel1_pp_1_1/emi_23';
 
if(o == e)
    assert(o_inv == e_inv, [emsg ' ; o_inv~=e_inv']);
    return;
end
 
if(o_inv > 0)
    assert(e_inv < 0, [emsg ' ; e_inv>=0']);
else
    assert(e_inv > 0, [emsg ' ; e_inv<=0']);
end

== matlab function sampleModel1_pp_1_1/emi_25 ==
  data: o input; e input
function  fcn(o, e)
o_inv = o^-1;
e_inv = e^-1;

emsg = 'sampleModel1_pp_1_1/emi_25';
 
if(o == e)
    assert(o_inv == e_inv, [emsg ' ; o_inv~=e_inv']);
    return;
end
 
if(o_inv > 0)
    assert(e_inv < 0, [emsg ' ; e_inv>=0']);
else
    assert(e_inv > 0, [emsg ' ; e_inv<=0']);
end

== matlab function sampleModel1_pp_1_1/emi_27 ==
  data: o input; e input
function  fcn(o, e)
o_inv = o^-1;
e_inv = e^-1;

emsg = 'sampleModel1_pp_1_1/emi_27';
 
if(o == e)
    assert(o_inv == e_inv, [emsg ' ; o_inv~=e_inv']);
    return;
end
 
if(o_inv > 0)
    assert(e_inv < 0, [emsg ' ; e_inv>=0']);
else
    assert(e_inv > 0, [emsg ' ; e_inv<=0']);
end
